simulink library "mc9s12tool"  (Simulink 7.4)
settings: Solver=ode45  SolverMode=SingleTasking  StartTime=0.0  StopTime=10.0  RelTol=1e-3
settings Model: Creator=Admin  LastModifiedBy=fw  ExtModeAutoUpdateStatusClock=off

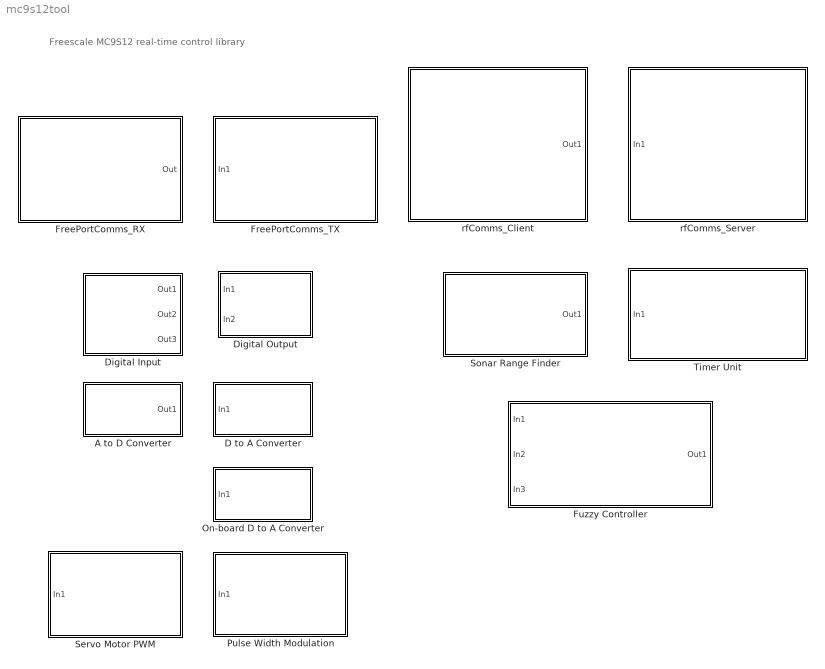
== system mc9s12tool ==
  note: Freescale MC9S12 real-time control library
  A to D Converter : Subsystem  Tag=mcTarget_adc  mask{bank=0, channels=2, use10bits=10 bits, normalize=max. output:  5, sampletime=0.01}
      mask prompts: bank "ADC bank"; channels "Channels ( 0 - 7 )"; use10bits "ADC resolution"; normalize "Normalization"; sampletime "Sample time"
      mask init:
      | [channelsStr, firstChannel, numChannels] = mbc_adcinput(channels);
      mask Help: web('adc_sfcn_9S12.html');
      mask StyleString: popup(0|1),edit,popup(10 bits|8 bits),popup(raw values|max. output:  1|max. output:  5),edit
      mask Display: disp(['A to D Converter\n' channelsStr])
  D to A Converter : Subsystem  Tag=mcTarget_dac  mask{sampletime=0.01, dac_channel=0, Vsat=5}
      mask prompts: sampletime "Sample time"; dac_channel "DAC channel"; Vsat "Saturation level (block input)"
      mask init:
      | % Check the sampletime value
      | if (sampletime < 0) | (sampletime > 3.355)
      |    fprintf ('DAC: Inadmissible sampletime value.\n');
      | end
      | 
      | % check saturation level
      | if(Vsat <= 0)
      | 	disp('DAC: Saturation level must be a postivie number. Assuming 5.')
      | 	Vsat = 5;
      | end
      | 
      | % channel numbers: 0, ...
      | dac_channel = dac_channel - 1;
      mask Help: web('dac_sfcn_9S12.html');
      mask StyleString: edit,popup(0|1),edit
      mask Display: fprintf('DAC%d\nVsat = %d', dac_channel, Vsat)
  Digital Input : Subsystem  Tag=mcTarget_digIn  mask{port=Port H, pin=0 1 2, sampletime=0.002}
      mask prompts: port "Port (see hardware manuals for valid options)"; pin "Pin (see hardware manuals for valid options)"; sampletime "Sample time"
      mask init:
      | [portstr, pinstr, pins] = mbc_digitalinput(port, pin, sampletime);
      mask Help: web('digIn_sfcn_9S12.html');
      mask StyleString: popup(Port A|Port B|Port H|Port J|Port M|Port P|Port S|Port T),edit,edit
      mask Display: fprintf('%s\nPins: %s', portstr, pinstr)
  Digital Output : Subsystem  Tag=mcTarget_digOut  mask{port=Port H, pin=2 6, sampletime=0.002, Von=3.5, Voff=2}
      mask prompts: port "Port (see hardware manuals for valid options)"; pin "Pin (see hardware manuals for valid options)"; sampletime "Sample time"; Von "On-threshold (Von)"; Voff "Off-threshold (Voff)"
      mask init:
      | [portstr, pinstr, pins] = mbc_digitaloutput(port, pin, sampletime, Von, Voff);
      mask Help: web('digOut_sfcn_9S12.html');
      mask StyleString: popup(Port A|Port B|Port H|Port J|Port M|Port P|Port S|Port T),edit,edit,edit,edit
      mask Display: fprintf('%s\nPins: %s', portstr, pinstr)
  FreePortComms_RX : Subsystem  Tag=mcTarget_freePortCommsRX  mask{sampletime=0.1, port=COM1, baudrate=115200, channel=0, buf_size=5, data_type=UINT8, format=off, outformat=on}
      mask prompts: sampletime "Sample time"; port "Communication port"; channel "Channel number"; buf_size "Number of elements"; data_type "Data Type"; format "Block receives raw data"; outformat "Block output is double"
      mask init:
      | [buf_sizestr, portNamestr, baudratestr, channelstr, data_type_str, sampletime_str] = mbc_freeportrxd(sampletime, port, baudrate, channel, buf_size, data_type, format, outformat);
      mask Help: web('freePortComms_rxd.html');
      mask StyleString: edit,popup(SCI0|SCI1|COM1|COM2|COM3|COM4),popup(300|600|1200|2400|4800|9600|19200|38400|57600|115200),edit,edit,popup(SINGLE|INT8|UINT8|INT16|UINT16|INT32|UINT32|BOOLEAN),checkbox,checkbox
      mask Display: fprintf('Receive %s element(s)\nComm port: %s\nBaudrate: %s bps\nChannel: %s\nData type: %s\n Sample rate: %s', buf_sizestr, portNamestr, baudratestr, channelstr, data_type_str, sampletime_str)
  FreePortComms_TX : Subsystem  Tag=mcTarget_freePortCommsTX  mask{sampletime=0.1, port=COM1, baudrate=115200, channel=0, buf_size=5, data_type=UINT8, format=off}
      mask prompts: sampletime "Sample time"; port "Communication port"; channel "Channel number"; buf_size "Number of elements"; data_type "Data Type"; format "Block sends raw data"
      mask init:
      | [buf_sizestr, portNamestr, baudratestr, channelstr, data_type_str, sampletime_str] = mbc_freeporttxd(sampletime, port, baudrate, channel, buf_size, data_type, format);
      mask Help: web('freePortComms_txd.html');
      mask StyleString: edit,popup(SCI0|SCI1|COM1|COM2|COM3|COM4),popup(300|600|1200|2400|4800|9600|19200|38400|57600|115200),edit,edit,popup(SINGLE|INT8|UINT8|INT16|UINT16|INT32|UINT32|BOOLEAN),checkbox
      mask Display: fprintf('Transmit %s element(s)\nComm port: %s\nBaudrate: %s bps\nChannel: %s\nData type: %s\n Sample rate: %s', buf_sizestr, portNamestr, baudratestr, channelstr, data_type_str, sampletime_str)
  Fuzzy Controller : Subsystem  Tag=mcTarget_fuzzy  mask{numInputs=3, MSFinput1=x1_3i1o.txt, MSFinput2=x2_3i1o.txt, MSFinput3=x3_3i1o.txt, MSFoutput=y_3i1o.txt, ruleBase=rb_3i1o.txt, sampletime=0.1}
      mask prompts: numInputs "Number of inputs"; MSFinput1 "MSFs input 1 (filename)"; MSFinput2 "MSFs input 2 (filename)"; MSFinput3 "MSFs input 3 (filename)"; MSFoutput "MSFs output (filename)"; ruleBase "Rule base (filename)"; sampletime "Sample time"
      mask init:
      | [MSFinputXstr, MSFoutputstr, ruleBasestr] = mbc_fuzzy(numInputs, MSFinput1, MSFinput2, MSFinput3, MSFoutput, ruleBase, sampletime);
      mask Help: web('fuzzy_ni1o.html');
      mask StyleString: popup(1|2|3),edit,edit,edit,edit,edit,edit
      mask Display: fprintf('%s\nMSFs output: %s\nRule base: %s', MSFinputXstr, MSFoutputstr, ruleBasestr)
  On-board D to A Converter : Subsystem  Tag=mcTarget_dacDragonOnBoard  mask{sampletime=0.01, dac_channel=0, Vsat=5}
      mask prompts: sampletime "Sample time"; dac_channel "DAC channel"; Vsat "Saturation level (block input)"
      mask init:
      | % Check the sampletime value
      | if (sampletime < 0) | (sampletime > 3.355)
      |    fprintf ('Onboard DAC: Inadmissible sampletime value.\n');
      | end
      | 
      | % check saturation level
      | if(Vsat <= 0)
      | 	disp('Onboard DAC: Saturation level must be a postivie number. Assuming 5.')
      | 	Vsat = 5;
      | end
      | 
      | % channel numbers: 0, ...
      | dac_channel = dac_channel - 1;
      mask Help: web('onboardDAC_sfcn_9S12.html');
      mask StyleString: edit,popup(0|1),edit
      mask Display: fprintf('DAC%d\nVsat = %d', dac_channel, Vsat)
  Pulse Width Modulation : Subsystem  Tag=mcTarget_pwm  mask{sampletime=0.01, resolution=16 bit, PWMperiod=2, pulse_pin=3  (8-bit / 16-bit), sign_port=PTH, sign_pin=4, Vmax=100, sig_mon=off}
      mask prompts: sampletime "Sample time"; PWMperiod "PWM period (8-bit : up to 0.699 s, 16-bit : up to 179 s)"; pulse_pin "Pulse pin (PTP)"; sign_port "Sign port"; sign_pin "Sign pin"; Vmax "Saturation input level [simulated voltage]"; sig_mon "Signal monitoring"
      mask init:
      | [pulsepinstr, signportstr, signpinstr, periodstr, clkABstr, resstr] = mbc_pwmoutput(sampletime, resolution, PWMperiod, pulse_pin, sign_port, sign_pin, Vmax, sig_mon);
      mask Help: web('pwm_sfcn_9S12.html');
      mask StyleString: edit,popup(8 bit|16 bit),edit,popup(0  (8-bit)|1  (8-bit / 16-bit)|2  (8-bit)|3  (8-bit / 16-bit)|4  (8-bit)|5  (8-bit / 16-bit)|6  (8-bit)|7  (8-bit / 16-bit)),popup(PORTA|PORTB|PTH|PTJ|PTM|PTP|PTT|PTS),popup(0|1|2|3|4|5|6|7),edit,checkbox
      mask Display: fprintf('PWM-%s, %s-bit\nPulse pin: PTP.%s\nSign pin: %s.%s\nPeriod: %s (s)\nSaturation: %d', clkABstr, resstr, pulsepinstr, signportstr, signpinstr, periodstr, Vmax)
  Servo Motor PWM : Subsystem  Tag=mcTarget_pwmServo  mask{sampletime=0.02, PWMperiod=0.02, minwidth=0.0006, maxwidth=0.0020, resolution=16 bit, pulse_pin=3  (8-bit / 16-bit), Vmax=1}
      mask prompts: sampletime "Sample time"; PWMperiod "PWM period (16-bit : up to 179 s)"; minwidth "Minimum pulse width"; maxwidth "Maximum pulse width"; pulse_pin "Pulse pin (PTP)"; Vmax "Saturation input level [simulated voltage]"
      mask init:
      | [pulsepinstr, periodstr, clkABstr, resolutionstr] = mbc_servopwmoutput(sampletime, PWMperiod, minwidth, maxwidth, resolution, pulse_pin, Vmax);
      mask Help: web('servo_pwm_sfcn_9S12.html');
      mask StyleString: edit,edit,edit,edit,popup(8 bit|16 bit),popup(0  (8-bit)|1  (8-bit / 16-bit)|2  (8-bit)|3  (8-bit / 16-bit)|4  (8-bit)|5  (8-bit / 16-bit)|6  (8-bit)|7  (8-bit / 16-bit)),edit
      mask Display: fprintf('Servo motor PWM\n(PWM clk: %s, %s-bit)\nPeriod: %s\nPulse pin: PTP.%s\nSaturation: %d', clkABstr, resolutionstr, periodstr, pulsepinstr, Vmax)
  Sonar Range Finder : Subsystem  Tag=mcTarget_sonar  mask{out_port=Port T, out_pin=0, in_port=Port T, in_pin=1, sampletime=0.02}
      mask prompts: out_port "Output port (trigger echo pulse train)"; out_pin "Output pin"; in_port "Input port (detect 'echo received')"; in_pin "Input pin"; sampletime "Sample time"
      mask init:
      | [out_portstr, out_pinstr, in_portstr, in_pinstr] = mbc_sonar(out_port, out_pin, in_port, in_pin, sampletime);
      mask Help: web('sonar_sfcn_9S12.html');
      mask StyleString: popup(Port A|Port B|Port H|Port J|Port M|Port P|Port S|Port T),popup(0|1|2|3|4|5|6|7),popup(Port A|Port B|Port H|Port J|Port M|Port P|Port S|Port T),popup(0|1|2|3|4|5|6|7),edit
      mask Display: fprintf('Output\n%s Pin %s\nInput\n%s Pin %s', out_portstr, out_pinstr, in_portstr, in_pinstr)
  Timer Unit : Subsystem  Tag=mcTarget_timer  mask{timerChannel=Channel 3, timerMode=Output Compare, timerPeriod=0.3, sampletime=0.1}
      mask prompts: timerChannel "Timer channel"; timerMode "Timer mode"; timerPeriod "Timer base period (seconds)"; sampletime "Sample time"
      mask init:
      | if(timerMode == 1)
      | 	% OC
      | 	timerPeriodTypestr = 'Period:';
      | else
      | 	% IC
      | 	timerPeriodTypestr = 'Measurement intvl:';
      | end
      | 
      | [timerChannelstr, timerModestr, timerPeriodstr, ECTResolutionstr] = mbc_timer(timerChannel, timerMode, timerPeriod, sampletime);
      | 
      | % future extension: allow for output port / pin selection
      | % this hasn't been implemented yet, as it would require the 
      | % interrupt service handlers to be configured by TLC
      | % fw-09-06
      | %
      | % the following code assumes that timerOCport and timerOCpin have been defined similarly to what's done in mbc_ditaloutput.m
      | % the function also returns two more parameters (timerPORTstr, timerPINstr)
      | % these can be used in the Icon page. Replace that line by the following:
      | % fprintf('Channel: %s\nMode: %s\n%sPeriod: %s\nResolution: %s', timerChannelstr, timerModestr, timerOptPORTstr, timerPeriodstr, ECTResolutionstr)
      | % 
      | % [timerChannelstr, timerModestr, timerPORTstr, timerPINstr, timerPeriodstr, ECTResolutionstr] = mbc_timer(timerChannel, timerMode, timerOCport, timerOCpin, timerPeriod, sampletime);
      | % 
      | % if(timerMode == 1)
      | % 	% OC -> display port / pin
      | % 	timerOptPORTstr = ['Toggle: ' timerPORTstr ', Pin(s): ' timerPINstr '\n'];
      | % else
      | % 	% IC -> don't display port / pin
      | % 	timerOptPORTstr = '';
      | % end
      mask Help: web('timer_sfcn_9S12.html');
      mask StyleString: popup(Channel 0|Channel 1|Channel 2|Channel 3|Channel 4|Channel 5|Channel 6),popup(Output Compare|Input Capture),edit,edit
      mask Display: fprintf('Channel: %s\nMode: %s\nPeriod: %s\nResolution: %s', timerChannelstr, timerModestr, timerPeriodstr, ECTResolutionstr)
  rfComms_Client : Subsystem  Tag=mcTarget_rfCommsCli  mask{sampletime=0.1, RXTXmode=Reception (RX), RFchannel=12, clientNum=1, serverAddress=0xe7e7e7e7, clientAddress=0xc2c2c2c2, channel=0, buf_size=1, data_type=UINT8, format=on, outformat=on}
      mask prompts: sampletime "Sample time"; RXTXmode "Communication mode (TX, RX)"; RFchannel "RF channel number (0 - 127)"; clientNum "Client number"; serverAddress "Server address (4 bytes, hexadecimal notation, e.g. 0xe7e7e7e7)"; clientAddress "Client address (4 bytes, hexadecimal notation, e.g.: 0xc2c2c2c2)"; channel "User channel number (0 - 9)"; buf_size "Number of elements to be sent/received"; data_type "Data Type"; format "Block sends/receives raw data"; outformat "Block output is 'double'"
      mask init:
      | [buf_sizestr, RXTXmodestr, RFchannelstr, clientstr, serverAddressstr, clientAddressstr, channelstr, data_type_str, sampletime_str] = mbc_rfComms_client(sampletime, RXTXmode, RFchannel, clientNum, serverAddress, clientAddress, channel, buf_size, data_type, format, outformat);
      mask Help: web('rfComms_client.html');
      mask StyleString: edit,popup(Reception (RX)|Transmission (TX)),edit,popup(1|2|3|4|5),edit,edit,edit,edit,popup(SINGLE|INT8|UINT8|INT16|UINT16|INT32|UINT32|BOOLEAN),checkbox,checkbox
      mask Display: fprintf('RF mode: %s\nRF channel: %s\nClient: %s\nServer address: %s\nClient address: %s\nUser channel: %s\nElements: %s\nData type: %s\n Sample rate: %s', RXTXmodestr, RFchannelstr, clientstr, serverAddressstr, clientAddressstr, channelstr, buf_sizestr, data_type_str, sampletime_str)
  rfComms_Server : Subsystem  Tag=mcTarget_rfCommsSrv  mask{sampletime=0.1, RXTXmode=Transmission (TX), RFchannel=12, numClient=1, serverAddress=0xe7e7e7e7, clientAddress=0xc2c2c2c2, channel=0, buf_size=5, data_type=UINT8, format=off, outformat=on}
      mask prompts: sampletime "Sample time"; RXTXmode "Communication mode (TX, RX)"; RFchannel "RF channel number (0 - 127)"; numClient "Client to transmit to"; serverAddress "Server address (4 bytes, hexadecimal notation, e.g. 0xe7e7e7e7)"; clientAddress "Client address (4 bytes, hexadecimal notation, e.g.: 0xc2c2c2c2)"; channel "User channel number (0 - 9)"; buf_size "Number of elements to be sent/received"; data_type "Data Type"; format "Block sends/receives raw data"; outformat "Block output is 'double'"
      mask init:
      | [buf_sizestr, RXTXmodestr, RFchannelstr, clientstr, serverAddressstr, clientAddressstr, channelstr, data_type_str, sampletime_str] = mbc_rfComms_server(sampletime, RXTXmode, RFchannel, numClient, serverAddress, clientAddress, channel, buf_size, data_type, format, outformat);
      mask Help: web('rfComms_server.html');
      mask StyleString: edit,popup(Reception (RX)|Transmission (TX)),edit,popup(1|2|3|4|5),edit,edit,edit,edit,popup(SINGLE|INT8|UINT8|INT16|UINT16|INT32|UINT32|BOOLEAN),checkbox,checkbox
      mask Display: fprintf('RF mode: %s\nRF channel: %s\n%s\nServer address: %s\nClient address: %s\nUser channel: %s\nElements: %s\nData type: %s\n Sample rate: %s', RXTXmodestr, RFchannelstr, clientstr, serverAddressstr, clientAddressstr, channelstr, buf_sizestr, data_type_str, sampletime_str)

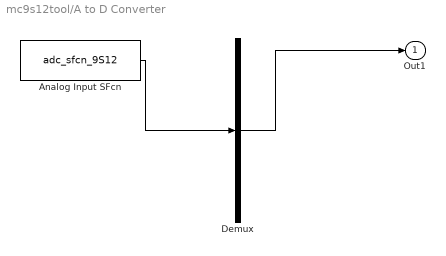
== system mc9s12tool/A to D Converter ==
  Analog Input SFcn : S-Function  Tag=mcTarget_adc  FunctionName=adc_sfcn_9S12  Parameters=bank-1, firstChannel, numChannels, use10bits-1, normalize, sampletime  EnableBusSupport=off
  Demux : Demux  Outputs=1
  Out1 : Outport  OutDataType=sfix(16)  OutScaling=2^0
  wires:
  Demux/1 -> Out1/1
  Analog Input SFcn/1 -> Demux/1

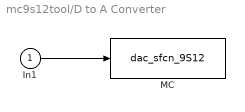
== system mc9s12tool/D to A Converter ==
  In1 : Inport  OutDataType=sfix(16)  OutScaling=2^0
  MC : S-Function  Tag=mcTarget_dac  FunctionName=dac_sfcn_9S12  Parameters=sampletime, dac_channel, Vsat  EnableBusSupport=off
  wires:
  In1/1 -> MC/1

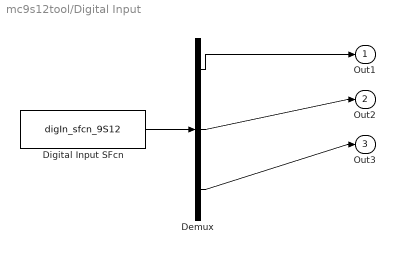
== system mc9s12tool/Digital Input ==
  Demux : Demux  Outputs=3
  Digital Input SFcn : S-Function  Tag=mcTarget_digIn  FunctionName=digIn_sfcn_9S12  Parameters=sampletime, port, pins  EnableBusSupport=off
  Out1 : Outport  OutDataType=sfix(16)  OutScaling=2^0
  Out2 : Outport  Port=2  OutDataType=sfix(16)  OutScaling=2^0
  Out3 : Outport  Port=3  OutDataType=sfix(16)  OutScaling=2^0
  wires:
  Digital Input SFcn/1 -> Demux/1
  Demux/1 -> Out1/1
  Demux/2 -> Out2/1
  Demux/3 -> Out3/1

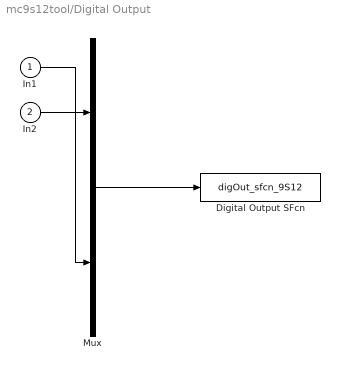
== system mc9s12tool/Digital Output ==
  In1 : Inport  OutDataType=sfix(16)  OutScaling=2^0
  In2 : Inport  Port=2  OutDataType=sfix(16)  OutScaling=2^0
  Digital Output SFcn : S-Function  Tag=mcTarget_digOut  FunctionName=digOut_sfcn_9S12  Parameters=sampletime, port, pins, Von, Voff  EnableBusSupport=off
  Mux : Mux  Inputs=2
  wires:
  Mux/1 -> Digital Output SFcn/1
  In1/1 -> Mux/1
  In2/1 -> Mux/2

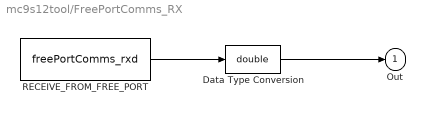
== system mc9s12tool/FreePortComms_RX ==
  Data Type Conversion : DataTypeConversion  OutDataTypeMode=double  OutDataType=sfix(16)  OutScaling=2^0  OutDataTypeStr=double  SaturateOnIntegerOverflow=on  RndMeth=Zero
  RECEIVE_FROM_FREE_PORT : S-Function  Tag=mcTarget_freePortCommsRX  FunctionName=freePortComms_rxd  Parameters=sampletime, channel, buf_size, data_type, port, baudrate, format  EnableBusSupport=off
  Out : Outport  OutDataType=sfix(16)  OutScaling=2^0
  wires:
  Data Type Conversion/1 -> Out/1
  RECEIVE_FROM_FREE_PORT/1 -> Data Type Conversion/1

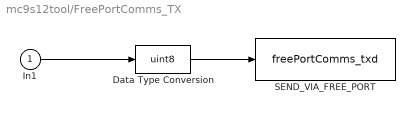
== system mc9s12tool/FreePortComms_TX ==
  In1 : Inport  OutDataType=sfix(16)  OutScaling=2^0
  Data Type Conversion : DataTypeConversion  OutDataTypeMode=uint8  OutDataType=sfix(16)  OutScaling=2^0  OutDataTypeStr=uint8  SaturateOnIntegerOverflow=on  RndMeth=Zero
  SEND_VIA_FREE_PORT : S-Function  Tag=mcTarget_freePortCommsTX  FunctionName=freePortComms_txd  Parameters=sampletime, channel, buf_size, data_type, port, baudrate, format  EnableBusSupport=off
  wires:
  Data Type Conversion/1 -> SEND_VIA_FREE_PORT/1
  In1/1 -> Data Type Conversion/1

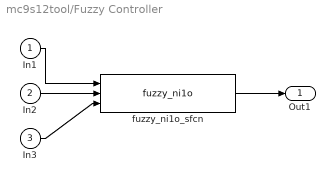
== system mc9s12tool/Fuzzy Controller ==
  In1 : Inport  OutDataType=sfix(16)  OutScaling=2^0
  In2 : Inport  Port=2  OutDataType=sfix(16)  OutScaling=2^0
  In3 : Inport  Port=3  OutDataType=sfix(16)  OutScaling=2^0
  fuzzy_ni1o_sfcn : S-Function  Tag=mcTarget_fuzzy  FunctionName=fuzzy_ni1o  Parameters=sampletime, numInputs  EnableBusSupport=off
  Out1 : Outport  OutDataType=sfix(16)  OutScaling=2^0
  wires:
  In3/1 -> fuzzy_ni1o_sfcn/3
  In2/1 -> fuzzy_ni1o_sfcn/2
  fuzzy_ni1o_sfcn/1 -> Out1/1
  In1/1 -> fuzzy_ni1o_sfcn/1

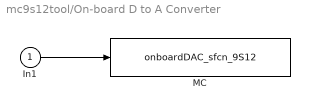
== system mc9s12tool/On-board D to A Converter ==
  In1 : Inport  OutDataType=sfix(16)  OutScaling=2^0
  MC : S-Function  Tag=mcTarget_dacDragonOnBoard  FunctionName=onboardDAC_sfcn_9S12  Parameters=sampletime, dac_channel, Vsat  EnableBusSupport=off
  wires:
  In1/1 -> MC/1

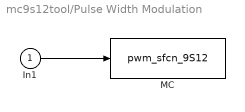
== system mc9s12tool/Pulse Width Modulation ==
  In1 : Inport  OutDataType=sfix(16)  OutScaling=2^0
  MC : S-Function  Tag=mcTarget_pwm  FunctionName=pwm_sfcn_9S12  Parameters=sampletime, PWMperiod, pulse_pin, sign_port, sign_pin, Vmax, sig_mon  EnableBusSupport=off
  wires:
  In1/1 -> MC/1

== system mc9s12tool/Servo Motor PWM ==
  In1 : Inport  OutDataType=sfix(16)  OutScaling=2^0
  servo pwm : S-Function  Tag=mcTarget_pwmServo  FunctionName=servo_pwm_sfcn_9S12  Parameters=sampletime, PWMperiod, pulse_pin, Vmax  EnableBusSupport=off
  wires:
  In1/1 -> servo pwm/1

== system mc9s12tool/Sonar Range Finder ==
  sonar pulse : S-Function  Tag=mcTarget_sonar  FunctionName=sonar_sfcn_9S12  Parameters=sampletime, out_port, out_pin, in_port, in_pin  EnableBusSupport=off
  Out1 : Outport  OutDataType=sfix(16)  OutScaling=2^0
  wires:
  sonar pulse/1 -> Out1/1

== system mc9s12tool/Timer Unit ==
  In1 : Inport  OutDataType=sfix(16)  OutScaling=2^0
  Timer Block : S-Function  Tag=mcTarget_timer  FunctionName=timer_sfcn_9S12  Parameters=sampletime, timerMode  EnableBusSupport=off
  wires:
  In1/1 -> Timer Block/1

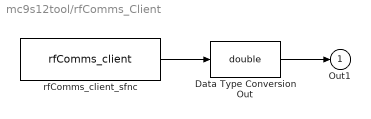
== system mc9s12tool/rfComms_Client ==
  Data Type Conversion Out : DataTypeConversion  OutDataTypeMode=double  OutDataType=sfix(16)  OutScaling=2^0  OutDataTypeStr=double  SaturateOnIntegerOverflow=on  RndMeth=Zero
  rfComms_client_sfnc : S-Function  Tag=mcTarget_rfCommsCli  FunctionName=rfComms_client  Parameters=sampletime, RXTXmode, channel, buf_size, data_type  EnableBusSupport=off
  Out1 : Outport  OutDataType=sfix(16)  OutScaling=2^0
  wires:
  rfComms_client_sfnc/1 -> Data Type Conversion Out/1
  Data Type Conversion Out/1 -> Out1/1

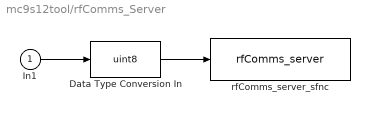
== system mc9s12tool/rfComms_Server ==
  In1 : Inport  OutDataType=sfix(16)  OutScaling=2^0
  Data Type Conversion In : DataTypeConversion  OutDataTypeMode=uint8  OutDataType=sfix(16)  OutScaling=2^0  OutDataTypeStr=uint8  SaturateOnIntegerOverflow=on  RndMeth=Zero
  rfComms_server_sfnc : S-Function  Tag=mcTarget_rfCommsSrv  FunctionName=rfComms_server  Parameters=sampletime, RXTXmode, channel, buf_size, data_type  EnableBusSupport=off
  wires:
  In1/1 -> Data Type Conversion In/1
  Data Type Conversion In/1 -> rfComms_server_sfnc/1
